simulink model "Q3"  (R2022a)
settings: Solver=VariableStepAuto  StartTime=0.0  StopTime=10  RelTol=1e-3
undefined symbols (not defined in the file): A, B, k123, k4
settings Model: Creator=ACER  LastModifiedBy=fatae
settings SolverCC: AlgebraicLoopSolver=TrustRegion
settings DataIOCC: ReturnWorkspaceOutputs=off
settings DebuggingCC: UnconnectedInputMsg=warning  UnconnectedOutputMsg=warning  UnconnectedLineMsg=warning  SFMachineParentedDataDiag=warning  ArithmeticOperatorsInVariantConditions=warning
settings SFSimCC: SimUseLocalCustomCode=off  CustomCodeUndefinedFunction=UseInterfaceOnly
settings RTWCC: RTWUseLocalCustomCode=off  DLArmComputeVersion=19.05

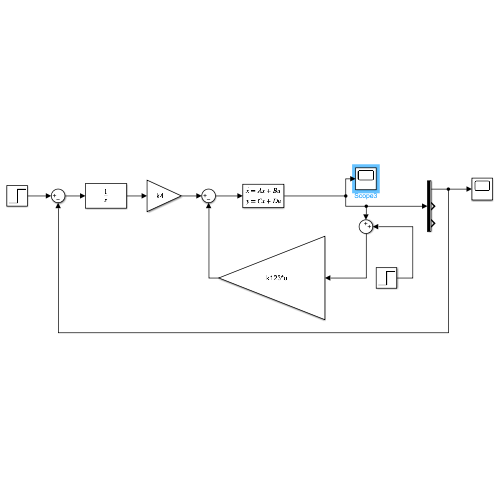
[thumbnail: Simulink's stored preview of the top-level diagram]
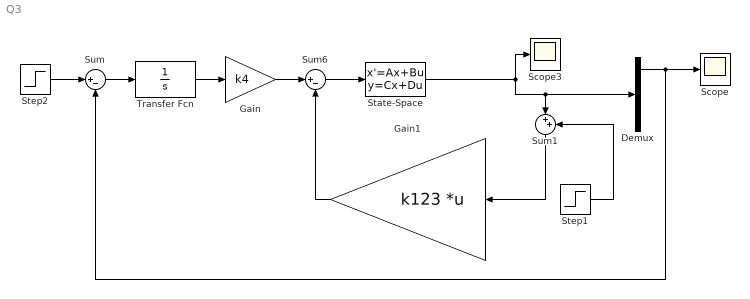
== system Q3 ==
  Demux : Demux  Outputs=3
  Gain : Gain  Gain=k4
  Gain1 : Gain  Gain=k123  Multiplication=Matrix(K*u)
  Scope : Scope
  Scope3 : Scope
  State-Space : StateSpace  A=A  B=B  C=eye(3)  D=[0;0;0]  InitialCondition=0
  Step1 : Step  After=0.2  SampleTime=0
  Step2 : Step  Time=0  SampleTime=0
  Sum : Sum  Inputs=|+-
  Sum1 : Sum  Inputs=|++
  Sum6 : Sum  Inputs=|+-
  Transfer Fcn : TransferFcn  Denominator=[1 0]
  wires:
  Gain1/1 -> Sum6/2
  State-Space/1 -> Sum1/1, Demux/1, Scope3/1
  Demux/1 -> Scope/1, Sum/2
  Sum6/1 -> State-Space/1
  Gain/1 -> Sum6/1
  Transfer Fcn/1 -> Gain/1
  Sum/1 -> Transfer Fcn/1
  Step2/1 -> Sum/1
  Sum1/1 -> Gain1/1
  Step1/1 -> Sum1/2
